simulink model "tema2_mdl2"  (R2019a)
settings: Solver=VariableStepAuto  StartTime=0.0  StopTime=400  RelTol=1e-3
values from neighbouring files (symbols this model uses):
  r = 2 * ystar    [tema2.m]
  Te = 0.06    [tema2.m]
settings Model: Creator=cynthia  LastModifiedBy=cynthia

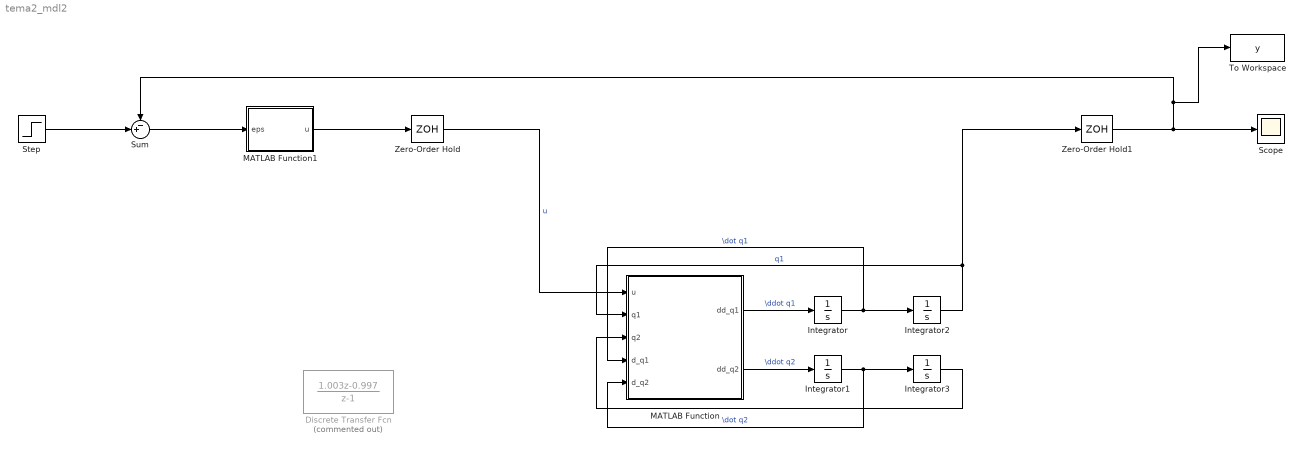
== system tema2_mdl2 ==
  Discrete Transfer Fcn : DiscreteTransferFcn  Commented=on  Numerator=[1.003 -0.997]  Denominator=[1 -1]
  Integrator{,1..3} (4 alike) : Integrator
  MATLAB Function : MATLAB Function  TreatAsAtomicUnit=on
  MATLAB Function1 : MATLAB Function  TreatAsAtomicUnit=on  SystemSampleTime=Te
  Scope : Scope
  Step : Step  Time=0  After=r  SampleTime=Te
  Sum : Sum  Inputs=-+|
  To Workspace : ToWorkspace  VariableName=y  SaveFormat=Timeseries  SampleTime=-1
  Zero-Order Hold : ZeroOrderHold  SampleTime=Te
  Zero-Order Hold1 : ZeroOrderHold  SampleTime=Te
  wires:
  MATLAB Function1/1(u) -> Zero-Order Hold/1
  Zero-Order Hold1/1 -> Sum/1, To Workspace/1, Scope/1
  Sum/1 -> MATLAB Function1/1(eps)
  Integrator3/1 -> MATLAB Function/3(q2)
  Integrator2/1 -> Zero-Order Hold1/1, MATLAB Function/2(q1)  "q1"
  MATLAB Function/1(dd_q1) -> Integrator/1  "\\ddot q1"
  MATLAB Function/2(dd_q2) -> Integrator1/1  "\\ddot q2"
  Integrator/1 -> Integrator2/1, MATLAB Function/4(d_q1)  "\\dot q1"
  Zero-Order Hold/1 -> MATLAB Function/1(u)  "u"
  Integrator1/1 -> Integrator3/1, MATLAB Function/5(d_q2)  "\\dot q2"
  Step/1 -> Sum/2

== matlab function tema2_mdl2/MATLAB Function1 ==
  data: eps input; u output
function u = fcn(eps)

persistent eps1; % eps[k-1]
persistent u1; % u[k-1]

if isempty(eps1)
    eps1 = 0 ;
end

if isempty(u1)
    u1 = 0;
end

%legea de comanda
% u[k] = u[k-1] + 1.003*eps[k] - 0.997*eps[k-1] 
u = u1 + 1.003 * eps - 0.997 * eps1;
u1 = u;
eps1 = eps;

== matlab function tema2_mdl2/MATLAB Function ==
  data: u input; dd_q1 output; q1 input; q2 input; d_q1 input; d_q2 input; dd_q2 output
function [dd_q1,dd_q2] = fcn(u,q1,q2,d_q1,d_q2)
m = 5.1;
g = 10;
L = 1.56;
zeta = 7.64;
k = 0.25;
J = 2.77; 
I = 1.89;
M = 2.82;

dd_q1 = (u + k*(q2-q1) - zeta*d_q1)/J;
dd_q2 = (-M*g*L*sin(q2) - k*(q2-q1) - zeta*d_q2)/I;


end
